simulink model "csc_est_state_estimation_hrn"  (R2014b)
settings: Solver=FixedStepDiscrete  StartTime=t0  StopTime=tFinal  FixedStep=sim_dt  RelTol=1e-3
libraries: util_common_lib x18, util_info_lib x1, csc_est_state_est_mtv_lib x1, csu_cfe_cfe_time_lib x1, converted_pressures_t_hrn_initialization x1, converted_temperatures_t_hrn_initialization x1
settings Model: Creator=escrane  LastModifiedBy=escrane
settings DebuggingCC: UnderspecifiedInitializationDetection=Classic  MergeDetectMultiDrivingBlocksExec=none  InheritedTsInSrcMsg=none

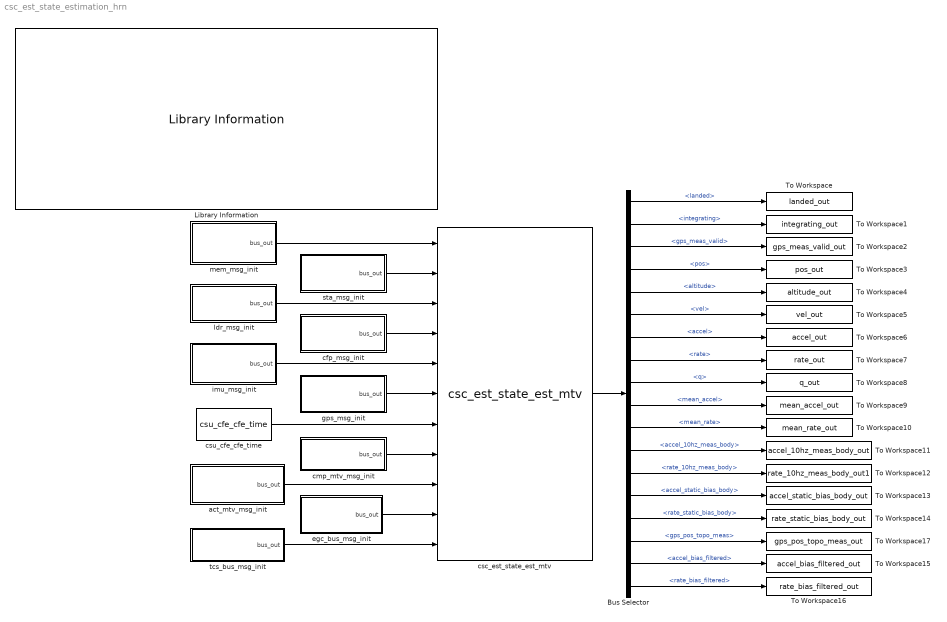
== system csc_est_state_estimation_hrn ==
  Bus Selector : BusSelector  OutputSignals=landed,integrating,gps_meas_valid,pos,altitude,vel,accel,rate,q,mean_accel,mean_rate,accel_10hz_meas_body,rate_10hz_meas_body,accel_static_bias_body,rate_static_bias_body,gps_pos_topo_meas,accel_bias_filtered,rate_bias_filtered
  Library Information : util_info_lib/Library Information  owner='escrane'
  To Workspace : ToWorkspace  VariableName=landed_out  SaveFormat=Timeseries  SampleTime=-1
  To Workspace1 : ToWorkspace  VariableName=integrating_out  SaveFormat=Timeseries  SampleTime=-1
  To Workspace10 : ToWorkspace  VariableName=mean_rate_out  SaveFormat=Timeseries  SampleTime=-1
  To Workspace11 : ToWorkspace  VariableName=accel_10hz_meas_body_out  SaveFormat=Timeseries  SampleTime=-1
  To Workspace12 : ToWorkspace  VariableName=rate_10hz_meas_body_out1  SaveFormat=Timeseries  SampleTime=-1
  To Workspace13 : ToWorkspace  VariableName=accel_static_bias_body_out  SaveFormat=Timeseries  SampleTime=-1
  To Workspace14 : ToWorkspace  VariableName=rate_static_bias_body_out  SaveFormat=Timeseries  SampleTime=-1
  To Workspace15 : ToWorkspace  VariableName=accel_bias_filtered_out  SaveFormat=Timeseries  SampleTime=-1
  To Workspace16 : ToWorkspace  VariableName=rate_bias_filtered_out  SaveFormat=Timeseries  SampleTime=-1
  To Workspace17 : ToWorkspace  VariableName=gps_pos_topo_meas_out  SaveFormat=Timeseries  SampleTime=-1
  To Workspace2 : ToWorkspace  VariableName=gps_meas_valid_out  SaveFormat=Timeseries  SampleTime=-1
  To Workspace3 : ToWorkspace  VariableName=pos_out  SaveFormat=Timeseries  SampleTime=-1
  To Workspace4 : ToWorkspace  VariableName=altitude_out  SaveFormat=Timeseries  SampleTime=-1
  To Workspace5 : ToWorkspace  VariableName=vel_out  SaveFormat=Timeseries  SampleTime=-1
  To Workspace6 : ToWorkspace  VariableName=accel_out  SaveFormat=Timeseries  SampleTime=-1
  To Workspace7 : ToWorkspace  VariableName=rate_out  SaveFormat=Timeseries  SampleTime=-1
  To Workspace8 : ToWorkspace  VariableName=q_out  SaveFormat=Timeseries  SampleTime=-1
  To Workspace9 : ToWorkspace  VariableName=mean_accel_out  SaveFormat=Timeseries  SampleTime=-1
  act_mtv_msg_init : Subsystem
  cfp_msg_init : Subsystem
  cmp_mtv_msg_init : Subsystem
  csc_est_state_est_mtv : csc_est_state_est_mtv_lib/csc_est_state_est_mtv  Tag=OFSW; MDL_TICK=CMP_MTV_MSG
  csu_cfe_cfe_time : csu_cfe_cfe_time_lib/csu_cfe_cfe_time  sch_dt=fsw_dt
  egc_bus_msg_init : Subsystem
  gps_msg_init : Subsystem
  imu_msg_init : Subsystem
  ldr_msg_init : Subsystem
  mem_msg_init : Subsystem
  sta_msg_init : Subsystem
  tcs_bus_msg_init : Subsystem
  wires:
  Bus Selector/1 -> To Workspace/1  "<landed>"
  csc_est_state_est_mtv/1 -> Bus Selector/1
  mem_msg_init/1(bus_out) -> csc_est_state_est_mtv/1
  cmp_mtv_msg_init/1(bus_out) -> csc_est_state_est_mtv/8
  act_mtv_msg_init/1(bus_out) -> csc_est_state_est_mtv/9
  gps_msg_init/1(bus_out) -> csc_est_state_est_mtv/6
  cfp_msg_init/1(bus_out) -> csc_est_state_est_mtv/4
  ldr_msg_init/1(bus_out) -> csc_est_state_est_mtv/3
  sta_msg_init/1(bus_out) -> csc_est_state_est_mtv/2
  csu_cfe_cfe_time/1 -> csc_est_state_est_mtv/7
  Bus Selector/2 -> To Workspace1/1  "<integrating>"
  Bus Selector/3 -> To Workspace2/1  "<gps_meas_valid>"
  Bus Selector/4 -> To Workspace3/1  "<pos>"
  Bus Selector/5 -> To Workspace4/1  "<altitude>"
  Bus Selector/6 -> To Workspace5/1  "<vel>"
  Bus Selector/7 -> To Workspace6/1  "<accel>"
  Bus Selector/8 -> To Workspace7/1  "<rate>"
  Bus Selector/9 -> To Workspace8/1  "<q>"
  Bus Selector/10 -> To Workspace9/1  "<mean_accel>"
  Bus Selector/11 -> To Workspace10/1  "<mean_rate>"
  Bus Selector/12 -> To Workspace11/1  "<accel_10hz_meas_body>"
  Bus Selector/13 -> To Workspace12/1  "<rate_10hz_meas_body>"
  Bus Selector/14 -> To Workspace13/1  "<accel_static_bias_body>"
  Bus Selector/15 -> To Workspace14/1  "<rate_static_bias_body>"
  Bus Selector/18 -> To Workspace16/1  "<rate_bias_filtered>"
  Bus Selector/17 -> To Workspace15/1  "<accel_bias_filtered>"
  Bus Selector/16 -> To Workspace17/1  "<gps_pos_topo_meas>"
  tcs_bus_msg_init/1(bus_out) -> csc_est_state_est_mtv/11
  egc_bus_msg_init/1(bus_out) -> csc_est_state_est_mtv/10
  imu_msg_init/1(bus_out) -> csc_est_state_est_mtv/5

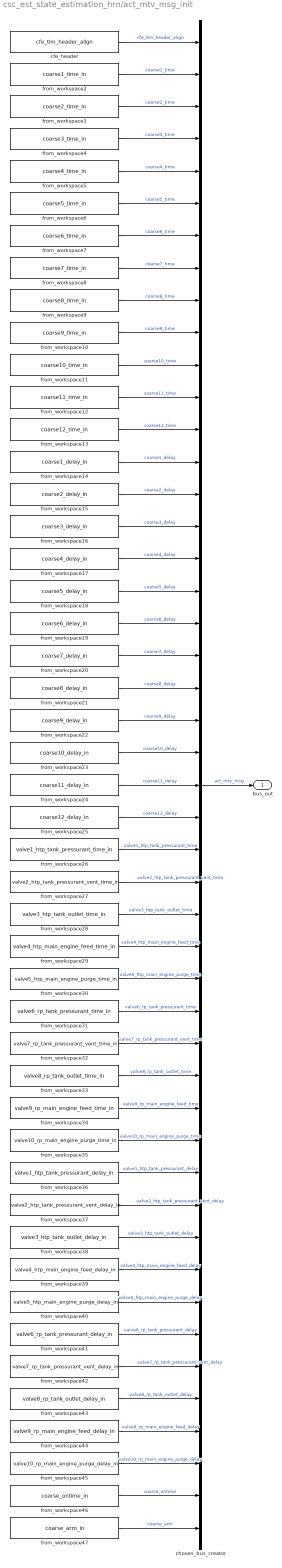
== system csc_est_state_estimation_hrn/act_mtv_msg_init ==
  cfe_header : util_common_lib/cfe_tlm_header_align
  chosen_bus_creator : BusCreator  Inputs=47  OutDataTypeStr=Bus: act_mtv_msg
  from_workspace10 : FromWorkspace  VariableName=coarse9_time_in
  from_workspace11 : FromWorkspace  VariableName=coarse10_time_in
  from_workspace12 : FromWorkspace  VariableName=coarse11_time_in
  from_workspace13 : FromWorkspace  VariableName=coarse12_time_in
  from_workspace14 : FromWorkspace  VariableName=coarse1_delay_in
  from_workspace15 : FromWorkspace  VariableName=coarse2_delay_in
  from_workspace16 : FromWorkspace  VariableName=coarse3_delay_in
  from_workspace17 : FromWorkspace  VariableName=coarse4_delay_in
  from_workspace18 : FromWorkspace  VariableName=coarse5_delay_in
  from_workspace19 : FromWorkspace  VariableName=coarse6_delay_in
  from_workspace2 : FromWorkspace  VariableName=coarse1_time_in
  from_workspace20 : FromWorkspace  VariableName=coarse7_delay_in
  from_workspace21 : FromWorkspace  VariableName=coarse8_delay_in
  from_workspace22 : FromWorkspace  VariableName=coarse9_delay_in
  from_workspace23 : FromWorkspace  VariableName=coarse10_delay_in
  from_workspace24 : FromWorkspace  VariableName=coarse11_delay_in
  from_workspace25 : FromWorkspace  VariableName=coarse12_delay_in
  from_workspace26 : FromWorkspace  VariableName=valve1_htp_tank_pressurant_time_in
  from_workspace27 : FromWorkspace  VariableName=valve2_htp_tank_pressurant_vent_time_in
  from_workspace28 : FromWorkspace  VariableName=valve3_htp_tank_outlet_time_in
  from_workspace29 : FromWorkspace  VariableName=valve4_htp_main_engine_feed_time_in
  from_workspace3 : FromWorkspace  VariableName=coarse2_time_in
  from_workspace30 : FromWorkspace  VariableName=valve5_htp_main_engine_purge_time_in
  from_workspace31 : FromWorkspace  VariableName=valve6_rp_tank_pressurant_time_in
  from_workspace32 : FromWorkspace  VariableName=valve7_rp_tank_pressurant_vent_time_in
  from_workspace33 : FromWorkspace  VariableName=valve8_rp_tank_outlet_time_in
  from_workspace34 : FromWorkspace  VariableName=valve9_rp_main_engine_feed_time_in
  from_workspace35 : FromWorkspace  VariableName=valve10_rp_main_engine_purge_time_in
  from_workspace36 : FromWorkspace  VariableName=valve1_htp_tank_pressurant_delay_in
  from_workspace37 : FromWorkspace  VariableName=valve2_htp_tank_pressurant_vent_delay_in
  from_workspace38 : FromWorkspace  VariableName=valve3_htp_tank_outlet_delay_in
  from_workspace39 : FromWorkspace  VariableName=valve4_htp_main_engine_feed_delay_in
  from_workspace4 : FromWorkspace  VariableName=coarse3_time_in
  from_workspace40 : FromWorkspace  VariableName=valve5_htp_main_engine_purge_delay_in
  from_workspace41 : FromWorkspace  VariableName=valve6_rp_tank_pressurant_delay_in
  from_workspace42 : FromWorkspace  VariableName=valve7_rp_tank_pressurant_vent_delay_in
  from_workspace43 : FromWorkspace  VariableName=valve8_rp_tank_outlet_delay_in
  from_workspace44 : FromWorkspace  VariableName=valve9_rp_main_engine_feed_delay_in
  from_workspace45 : FromWorkspace  VariableName=valve10_rp_main_engine_purge_delay_in
  from_workspace46 : FromWorkspace  VariableName=coarse_ontime_in
  from_workspace47 : FromWorkspace  VariableName=coarse_arm_in
  from_workspace5 : FromWorkspace  VariableName=coarse4_time_in
  from_workspace6 : FromWorkspace  VariableName=coarse5_time_in
  from_workspace7 : FromWorkspace  VariableName=coarse6_time_in
  from_workspace8 : FromWorkspace  VariableName=coarse7_time_in
  from_workspace9 : FromWorkspace  VariableName=coarse8_time_in
  bus_out : Outport
  wires:
  from_workspace47/1 -> chosen_bus_creator/47  "coarse_arm"
  from_workspace46/1 -> chosen_bus_creator/46  "coarse_ontime"
  from_workspace45/1 -> chosen_bus_creator/45  "valve10_rp_main_engine_purge_delay"
  from_workspace44/1 -> chosen_bus_creator/44  "valve9_rp_main_engine_feed_delay"
  from_workspace43/1 -> chosen_bus_creator/43  "valve8_rp_tank_outlet_delay"
  from_workspace42/1 -> chosen_bus_creator/42  "valve7_rp_tank_pressurant_vent_delay"
  from_workspace41/1 -> chosen_bus_creator/41  "valve6_rp_tank_pressurant_delay"
  from_workspace40/1 -> chosen_bus_creator/40  "valve5_htp_main_engine_purge_delay"
  from_workspace39/1 -> chosen_bus_creator/39  "valve4_htp_main_engine_feed_delay"
  from_workspace38/1 -> chosen_bus_creator/38  "valve3_htp_tank_outlet_delay"
  from_workspace37/1 -> chosen_bus_creator/37  "valve2_htp_tank_pressurant_vent_delay"
  from_workspace36/1 -> chosen_bus_creator/36  "valve1_htp_tank_pressurant_delay"
  from_workspace35/1 -> chosen_bus_creator/35  "valve10_rp_main_engine_purge_time"
  from_workspace34/1 -> chosen_bus_creator/34  "valve9_rp_main_engine_feed_time"
  from_workspace33/1 -> chosen_bus_creator/33  "valve8_rp_tank_outlet_time"
  from_workspace32/1 -> chosen_bus_creator/32  "valve7_rp_tank_pressurant_vent_time"
  from_workspace31/1 -> chosen_bus_creator/31  "valve6_rp_tank_pressurant_time"
  from_workspace30/1 -> chosen_bus_creator/30  "valve5_htp_main_engine_purge_time"
  from_workspace29/1 -> chosen_bus_creator/29  "valve4_htp_main_engine_feed_time"
  from_workspace28/1 -> chosen_bus_creator/28  "valve3_htp_tank_outlet_time"
  from_workspace27/1 -> chosen_bus_creator/27  "valve2_htp_tank_pressurant_vent_time"
  from_workspace26/1 -> chosen_bus_creator/26  "valve1_htp_tank_pressurant_time"
  from_workspace25/1 -> chosen_bus_creator/25  "coarse12_delay"
  from_workspace24/1 -> chosen_bus_creator/24  "coarse11_delay"
  from_workspace23/1 -> chosen_bus_creator/23  "coarse10_delay"
  from_workspace22/1 -> chosen_bus_creator/22  "coarse9_delay"
  from_workspace21/1 -> chosen_bus_creator/21  "coarse8_delay"
  from_workspace20/1 -> chosen_bus_creator/20  "coarse7_delay"
  from_workspace19/1 -> chosen_bus_creator/19  "coarse6_delay"
  from_workspace18/1 -> chosen_bus_creator/18  "coarse5_delay"
  from_workspace17/1 -> chosen_bus_creator/17  "coarse4_delay"
  from_workspace16/1 -> chosen_bus_creator/16  "coarse3_delay"
  from_workspace15/1 -> chosen_bus_creator/15  "coarse2_delay"
  from_workspace14/1 -> chosen_bus_creator/14  "coarse1_delay"
  from_workspace13/1 -> chosen_bus_creator/13  "coarse12_time"
  from_workspace12/1 -> chosen_bus_creator/12  "coarse11_time"
  from_workspace11/1 -> chosen_bus_creator/11  "coarse10_time"
  from_workspace10/1 -> chosen_bus_creator/10  "coarse9_time"
  from_workspace9/1 -> chosen_bus_creator/9  "coarse8_time"
  from_workspace8/1 -> chosen_bus_creator/8  "coarse7_time"
  from_workspace7/1 -> chosen_bus_creator/7  "coarse6_time"
  from_workspace6/1 -> chosen_bus_creator/6  "coarse5_time"
  from_workspace5/1 -> chosen_bus_creator/5  "coarse4_time"
  from_workspace4/1 -> chosen_bus_creator/4  "coarse3_time"
  from_workspace3/1 -> chosen_bus_creator/3  "coarse2_time"
  from_workspace2/1 -> chosen_bus_creator/2  "coarse1_time"
  cfe_header/1 -> chosen_bus_creator/1  "cfe_tlm_header_align"
  chosen_bus_creator/1 -> bus_out/1  "act_mtv_msg"

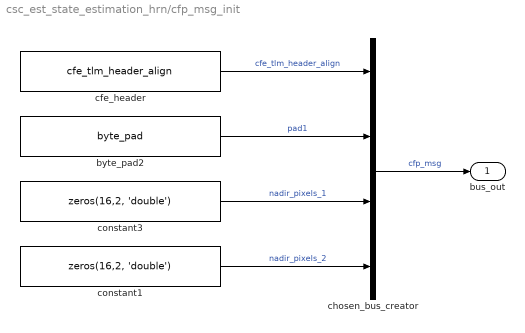
== system csc_est_state_estimation_hrn/cfp_msg_init ==
  byte_pad2 : util_common_lib/byte_pad  n_bytes=4
  cfe_header : util_common_lib/cfe_tlm_header_align
  chosen_bus_creator : BusCreator  OutDataTypeStr=Bus: cfp_msg  NonVirtualBus=on
  constant1 : Constant  Value=zeros(16,2, 'double')
  constant3 : Constant  Value=zeros(16,2, 'double')
  bus_out : Outport
  wires:
  constant1/1 -> chosen_bus_creator/4  "nadir_pixels_2"
  constant3/1 -> chosen_bus_creator/3  "nadir_pixels_1"
  byte_pad2/1 -> chosen_bus_creator/2  "pad1"
  cfe_header/1 -> chosen_bus_creator/1  "cfe_tlm_header_align"
  chosen_bus_creator/1 -> bus_out/1  "cfp_msg"

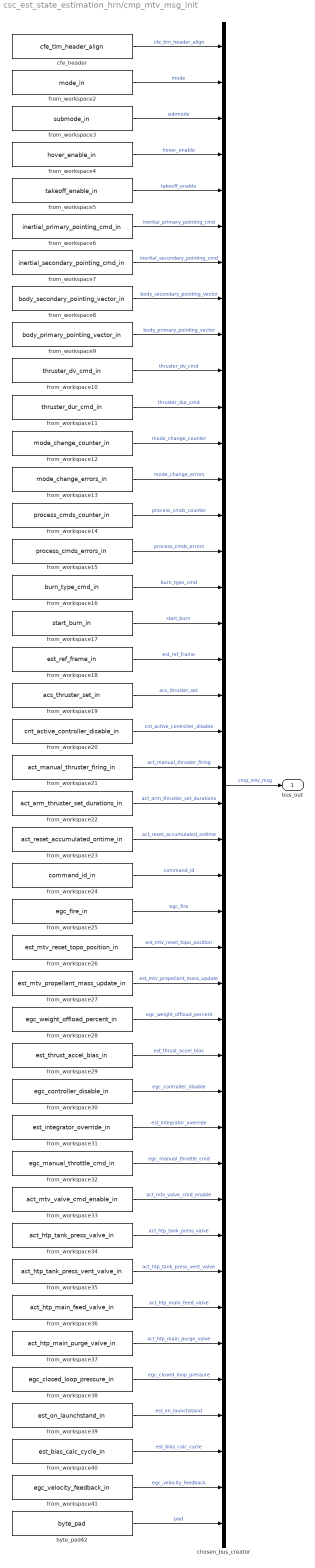
== system csc_est_state_estimation_hrn/cmp_mtv_msg_init ==
  byte_pad42 : util_common_lib/byte_pad  n_bytes=1
  cfe_header : util_common_lib/cfe_tlm_header_align
  chosen_bus_creator : BusCreator  Inputs=42  OutDataTypeStr=Bus: cmp_mtv_msg  NonVirtualBus=on
  from_workspace10 : FromWorkspace  VariableName=thruster_dv_cmd_in
  from_workspace11 : FromWorkspace  VariableName=thruster_dur_cmd_in
  from_workspace12 : FromWorkspace  VariableName=mode_change_counter_in
  from_workspace13 : FromWorkspace  VariableName=mode_change_errors_in
  from_workspace14 : FromWorkspace  VariableName=process_cmds_counter_in
  from_workspace15 : FromWorkspace  VariableName=process_cmds_errors_in
  from_workspace16 : FromWorkspace  VariableName=burn_type_cmd_in
  from_workspace17 : FromWorkspace  VariableName=start_burn_in
  from_workspace18 : FromWorkspace  VariableName=est_ref_frame_in
  from_workspace19 : FromWorkspace  VariableName=acs_thruster_set_in
  from_workspace2 : FromWorkspace  VariableName=mode_in
  from_workspace20 : FromWorkspace  VariableName=cnt_active_controller_disable_in
  from_workspace21 : FromWorkspace  VariableName=act_manual_thruster_firing_in
  from_workspace22 : FromWorkspace  VariableName=act_arm_thruster_set_durations_in
  from_workspace23 : FromWorkspace  VariableName=act_reset_accumulated_ontime_in
  from_workspace24 : FromWorkspace  VariableName=command_id_in
  from_workspace25 : FromWorkspace  VariableName=egc_fire_in
  from_workspace26 : FromWorkspace  VariableName=est_mtv_reset_topo_position_in
  from_workspace27 : FromWorkspace  VariableName=est_mtv_propellant_mass_update_in
  from_workspace28 : FromWorkspace  VariableName=egc_weight_offload_percent_in
  from_workspace29 : FromWorkspace  VariableName=est_thrust_accel_bias_in
  from_workspace3 : FromWorkspace  VariableName=submode_in
  from_workspace30 : FromWorkspace  VariableName=egc_controller_disable_in
  from_workspace31 : FromWorkspace  VariableName=est_integrator_override_in
  from_workspace32 : FromWorkspace  VariableName=egc_manual_throttle_cmd_in
  from_workspace33 : FromWorkspace  VariableName=act_mtv_valve_cmd_enable_in
  from_workspace34 : FromWorkspace  VariableName=act_htp_tank_press_valve_in
  from_workspace35 : FromWorkspace  VariableName=act_htp_tank_press_vent_valve_in
  from_workspace36 : FromWorkspace  VariableName=act_htp_main_feed_valve_in
  from_workspace37 : FromWorkspace  VariableName=act_htp_main_purge_valve_in
  from_workspace38 : FromWorkspace  VariableName=egc_closed_loop_pressure_in
  from_workspace39 : FromWorkspace  VariableName=est_on_launchstand_in
  from_workspace4 : FromWorkspace  VariableName=hover_enable_in
  from_workspace40 : FromWorkspace  VariableName=est_bias_calc_cycle_in
  from_workspace41 : FromWorkspace  VariableName=egc_velocity_feedback_in
  from_workspace5 : FromWorkspace  VariableName=takeoff_enable_in
  from_workspace6 : FromWorkspace  VariableName=inertial_primary_pointing_cmd_in
  from_workspace7 : FromWorkspace  VariableName=inertial_secondary_pointing_cmd_in
  from_workspace8 : FromWorkspace  VariableName=body_secondary_pointing_vector_in
  from_workspace9 : FromWorkspace  VariableName=body_primary_pointing_vector_in
  bus_out : Outport
  wires:
  byte_pad42/1 -> chosen_bus_creator/42  "pad"
  from_workspace41/1 -> chosen_bus_creator/41  "egc_velocity_feedback"
  from_workspace40/1 -> chosen_bus_creator/40  "est_bias_calc_cycle"
  from_workspace39/1 -> chosen_bus_creator/39  "est_on_launchstand"
  from_workspace38/1 -> chosen_bus_creator/38  "egc_closed_loop_pressure"
  from_workspace37/1 -> chosen_bus_creator/37  "act_htp_main_purge_valve"
  from_workspace36/1 -> chosen_bus_creator/36  "act_htp_main_feed_valve"
  from_workspace35/1 -> chosen_bus_creator/35  "act_htp_tank_press_vent_valve"
  from_workspace34/1 -> chosen_bus_creator/34  "act_htp_tank_press_valve"
  from_workspace33/1 -> chosen_bus_creator/33  "act_mtv_valve_cmd_enable"
  from_workspace32/1 -> chosen_bus_creator/32  "egc_manual_throttle_cmd"
  from_workspace31/1 -> chosen_bus_creator/31  "est_integrator_override"
  from_workspace30/1 -> chosen_bus_creator/30  "egc_controller_disable"
  from_workspace29/1 -> chosen_bus_creator/29  "est_thrust_accel_bias"
  from_workspace28/1 -> chosen_bus_creator/28  "egc_weight_offload_percent"
  from_workspace27/1 -> chosen_bus_creator/27  "est_mtv_propellant_mass_update"
  from_workspace26/1 -> chosen_bus_creator/26  "est_mtv_reset_topo_position"
  from_workspace25/1 -> chosen_bus_creator/25  "egc_fire"
  from_workspace24/1 -> chosen_bus_creator/24  "command_id"
  from_workspace23/1 -> chosen_bus_creator/23  "act_reset_accumulated_ontime"
  from_workspace22/1 -> chosen_bus_creator/22  "act_arm_thruster_set_durations"
  from_workspace21/1 -> chosen_bus_creator/21  "act_manual_thruster_firing"
  from_workspace20/1 -> chosen_bus_creator/20  "cnt_active_controller_disable"
  from_workspace19/1 -> chosen_bus_creator/19  "acs_thruster_set"
  from_workspace18/1 -> chosen_bus_creator/18  "est_ref_frame"
  from_workspace17/1 -> chosen_bus_creator/17  "start_burn"
  from_workspace16/1 -> chosen_bus_creator/16  "burn_type_cmd"
  from_workspace15/1 -> chosen_bus_creator/15  "process_cmds_errors"
  from_workspace14/1 -> chosen_bus_creator/14  "process_cmds_counter"
  from_workspace13/1 -> chosen_bus_creator/13  "mode_change_errors"
  from_workspace12/1 -> chosen_bus_creator/12  "mode_change_counter"
  from_workspace11/1 -> chosen_bus_creator/11  "thruster_dur_cmd"
  from_workspace10/1 -> chosen_bus_creator/10  "thruster_dv_cmd"
  from_workspace9/1 -> chosen_bus_creator/9  "body_primary_pointing_vector"
  from_workspace8/1 -> chosen_bus_creator/8  "body_secondary_pointing_vector"
  from_workspace7/1 -> chosen_bus_creator/7  "inertial_secondary_pointing_cmd"
  from_workspace6/1 -> chosen_bus_creator/6  "inertial_primary_pointing_cmd"
  from_workspace5/1 -> chosen_bus_creator/5  "takeoff_enable"
  from_workspace4/1 -> chosen_bus_creator/4  "hover_enable"
  from_workspace3/1 -> chosen_bus_creator/3  "submode"
  from_workspace2/1 -> chosen_bus_creator/2  "mode"
  cfe_header/1 -> chosen_bus_creator/1  "cfe_tlm_header_align"
  chosen_bus_creator/1 -> bus_out/1  "cmp_mtv_msg"

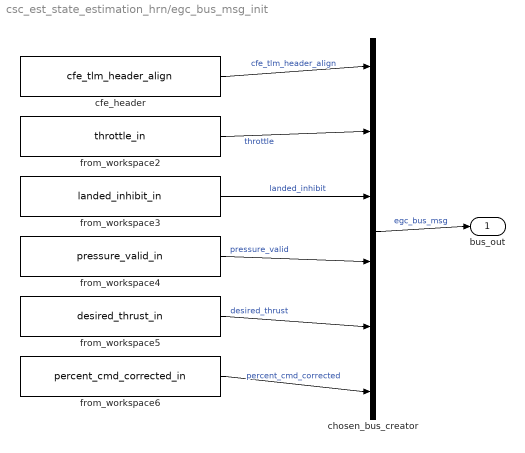
== system csc_est_state_estimation_hrn/egc_bus_msg_init ==
  cfe_header : util_common_lib/cfe_tlm_header_align
  chosen_bus_creator : BusCreator  Inputs=6  OutDataTypeStr=Bus: egc_bus_msg  NonVirtualBus=on
  from_workspace2 : FromWorkspace  VariableName=throttle_in
  from_workspace3 : FromWorkspace  VariableName=landed_inhibit_in
  from_workspace4 : FromWorkspace  VariableName=pressure_valid_in
  from_workspace5 : FromWorkspace  VariableName=desired_thrust_in
  from_workspace6 : FromWorkspace  VariableName=percent_cmd_corrected_in
  bus_out : Outport
  wires:
  from_workspace6/1 -> chosen_bus_creator/6  "percent_cmd_corrected"
  from_workspace5/1 -> chosen_bus_creator/5  "desired_thrust"
  from_workspace4/1 -> chosen_bus_creator/4  "pressure_valid"
  from_workspace3/1 -> chosen_bus_creator/3  "landed_inhibit"
  from_workspace2/1 -> chosen_bus_creator/2  "throttle"
  cfe_header/1 -> chosen_bus_creator/1  "cfe_tlm_header_align"
  chosen_bus_creator/1 -> bus_out/1  "egc_bus_msg"

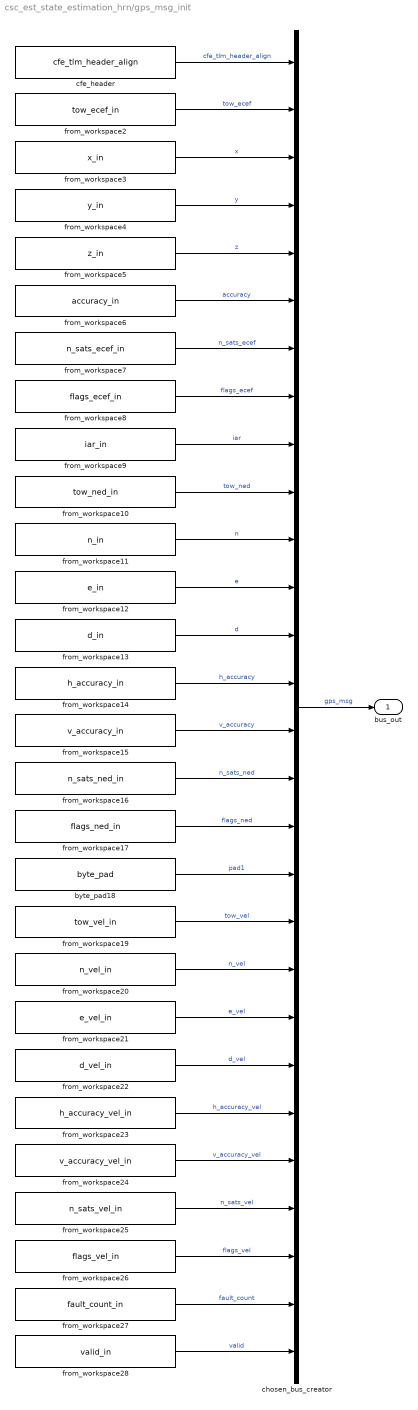
== system csc_est_state_estimation_hrn/gps_msg_init ==
  byte_pad18 : util_common_lib/byte_pad  n_bytes=2
  cfe_header : util_common_lib/cfe_tlm_header_align
  chosen_bus_creator : BusCreator  Inputs=28  OutDataTypeStr=Bus: gps_msg  NonVirtualBus=on
  from_workspace10 : FromWorkspace  VariableName=tow_ned_in
  from_workspace11 : FromWorkspace  VariableName=n_in
  from_workspace12 : FromWorkspace  VariableName=e_in
  from_workspace13 : FromWorkspace  VariableName=d_in
  from_workspace14 : FromWorkspace  VariableName=h_accuracy_in
  from_workspace15 : FromWorkspace  VariableName=v_accuracy_in
  from_workspace16 : FromWorkspace  VariableName=n_sats_ned_in
  from_workspace17 : FromWorkspace  VariableName=flags_ned_in
  from_workspace19 : FromWorkspace  VariableName=tow_vel_in
  from_workspace2 : FromWorkspace  VariableName=tow_ecef_in
  from_workspace20 : FromWorkspace  VariableName=n_vel_in
  from_workspace21 : FromWorkspace  VariableName=e_vel_in
  from_workspace22 : FromWorkspace  VariableName=d_vel_in
  from_workspace23 : FromWorkspace  VariableName=h_accuracy_vel_in
  from_workspace24 : FromWorkspace  VariableName=v_accuracy_vel_in
  from_workspace25 : FromWorkspace  VariableName=n_sats_vel_in
  from_workspace26 : FromWorkspace  VariableName=flags_vel_in
  from_workspace27 : FromWorkspace  VariableName=fault_count_in
  from_workspace28 : FromWorkspace  VariableName=valid_in
  from_workspace3 : FromWorkspace  VariableName=x_in
  from_workspace4 : FromWorkspace  VariableName=y_in
  from_workspace5 : FromWorkspace  VariableName=z_in
  from_workspace6 : FromWorkspace  VariableName=accuracy_in
  from_workspace7 : FromWorkspace  VariableName=n_sats_ecef_in
  from_workspace8 : FromWorkspace  VariableName=flags_ecef_in
  from_workspace9 : FromWorkspace  VariableName=iar_in
  bus_out : Outport
  wires:
  from_workspace28/1 -> chosen_bus_creator/28  "valid"
  from_workspace27/1 -> chosen_bus_creator/27  "fault_count"
  from_workspace26/1 -> chosen_bus_creator/26  "flags_vel"
  from_workspace25/1 -> chosen_bus_creator/25  "n_sats_vel"
  from_workspace24/1 -> chosen_bus_creator/24  "v_accuracy_vel"
  from_workspace23/1 -> chosen_bus_creator/23  "h_accuracy_vel"
  from_workspace22/1 -> chosen_bus_creator/22  "d_vel"
  from_workspace21/1 -> chosen_bus_creator/21  "e_vel"
  from_workspace20/1 -> chosen_bus_creator/20  "n_vel"
  from_workspace19/1 -> chosen_bus_creator/19  "tow_vel"
  byte_pad18/1 -> chosen_bus_creator/18  "pad1"
  from_workspace17/1 -> chosen_bus_creator/17  "flags_ned"
  from_workspace16/1 -> chosen_bus_creator/16  "n_sats_ned"
  from_workspace15/1 -> chosen_bus_creator/15  "v_accuracy"
  from_workspace14/1 -> chosen_bus_creator/14  "h_accuracy"
  from_workspace13/1 -> chosen_bus_creator/13  "d"
  from_workspace12/1 -> chosen_bus_creator/12  "e"
  from_workspace11/1 -> chosen_bus_creator/11  "n"
  from_workspace10/1 -> chosen_bus_creator/10  "tow_ned"
  from_workspace9/1 -> chosen_bus_creator/9  "iar"
  from_workspace8/1 -> chosen_bus_creator/8  "flags_ecef"
  from_workspace7/1 -> chosen_bus_creator/7  "n_sats_ecef"
  from_workspace6/1 -> chosen_bus_creator/6  "accuracy"
  from_workspace5/1 -> chosen_bus_creator/5  "z"
  from_workspace4/1 -> chosen_bus_creator/4  "y"
  from_workspace3/1 -> chosen_bus_creator/3  "x"
  from_workspace2/1 -> chosen_bus_creator/2  "tow_ecef"
  cfe_header/1 -> chosen_bus_creator/1  "cfe_tlm_header_align"
  chosen_bus_creator/1 -> bus_out/1  "gps_msg"

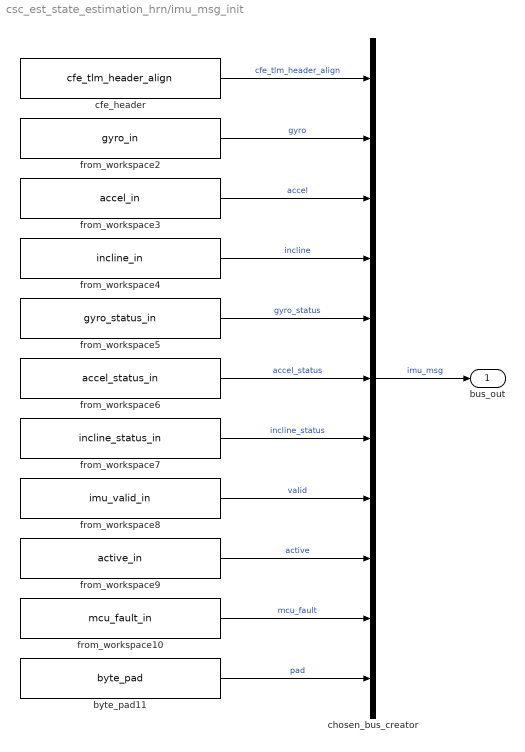
== system csc_est_state_estimation_hrn/imu_msg_init ==
  byte_pad11 : util_common_lib/byte_pad  n_bytes=2
  cfe_header : util_common_lib/cfe_tlm_header_align
  chosen_bus_creator : BusCreator  Inputs=11  OutDataTypeStr=Bus: imu_msg  NonVirtualBus=on
  from_workspace10 : FromWorkspace  VariableName=mcu_fault_in
  from_workspace2 : FromWorkspace  VariableName=gyro_in
  from_workspace3 : FromWorkspace  VariableName=accel_in
  from_workspace4 : FromWorkspace  VariableName=incline_in
  from_workspace5 : FromWorkspace  VariableName=gyro_status_in
  from_workspace6 : FromWorkspace  VariableName=accel_status_in
  from_workspace7 : FromWorkspace  VariableName=incline_status_in
  from_workspace8 : FromWorkspace  VariableName=imu_valid_in
  from_workspace9 : FromWorkspace  VariableName=active_in
  bus_out : Outport
  wires:
  byte_pad11/1 -> chosen_bus_creator/11  "pad"
  from_workspace10/1 -> chosen_bus_creator/10  "mcu_fault"
  from_workspace9/1 -> chosen_bus_creator/9  "active"
  from_workspace8/1 -> chosen_bus_creator/8  "valid"
  from_workspace7/1 -> chosen_bus_creator/7  "incline_status"
  from_workspace6/1 -> chosen_bus_creator/6  "accel_status"
  from_workspace5/1 -> chosen_bus_creator/5  "gyro_status"
  from_workspace4/1 -> chosen_bus_creator/4  "incline"
  from_workspace3/1 -> chosen_bus_creator/3  "accel"
  from_workspace2/1 -> chosen_bus_creator/2  "gyro"
  cfe_header/1 -> chosen_bus_creator/1  "cfe_tlm_header_align"
  chosen_bus_creator/1 -> bus_out/1  "imu_msg"

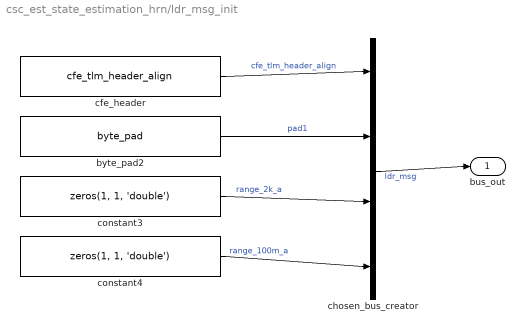
== system csc_est_state_estimation_hrn/ldr_msg_init ==
  byte_pad2 : util_common_lib/byte_pad  n_bytes=4
  cfe_header : util_common_lib/cfe_tlm_header_align
  chosen_bus_creator : BusCreator  OutDataTypeStr=Bus: ldr_msg  NonVirtualBus=on
  constant3 : Constant  Value=zeros(1, 1, 'double')
  constant4 : Constant  Value=zeros(1, 1, 'double')
  bus_out : Outport
  wires:
  constant4/1 -> chosen_bus_creator/4  "range_100m_a"
  constant3/1 -> chosen_bus_creator/3  "range_2k_a"
  byte_pad2/1 -> chosen_bus_creator/2  "pad1"
  cfe_header/1 -> chosen_bus_creator/1  "cfe_tlm_header_align"
  chosen_bus_creator/1 -> bus_out/1  "ldr_msg"

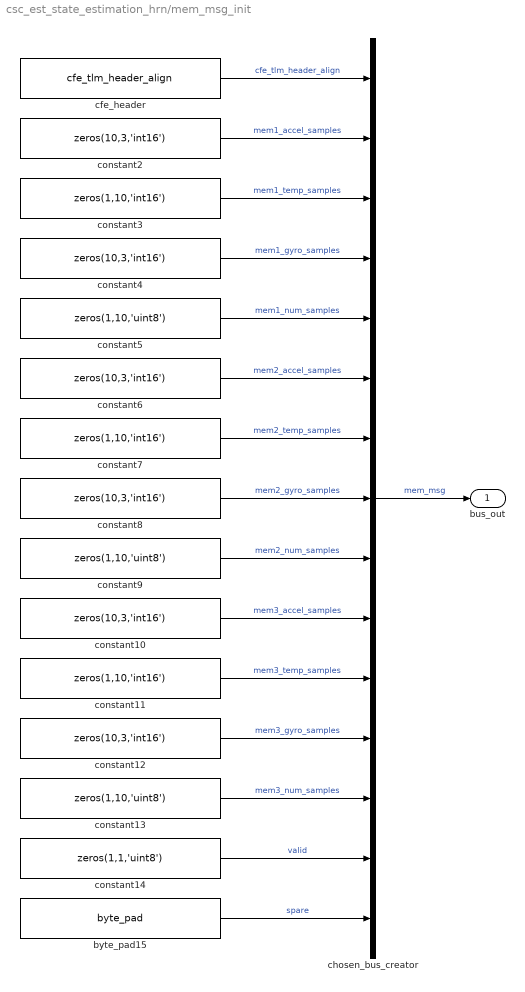
== system csc_est_state_estimation_hrn/mem_msg_init ==
  byte_pad15 : util_common_lib/byte_pad  n_bytes=1
  cfe_header : util_common_lib/cfe_tlm_header_align
  chosen_bus_creator : BusCreator  Inputs=15  OutDataTypeStr=Bus: mem_msg  NonVirtualBus=on
  constant{2,4,6,8,10,12} (6 alike) : Constant  Value=zeros(10,3,'int16')
  constant11 : Constant  Value=zeros(1,10,'int16')
  constant13 : Constant  Value=zeros(1,10,'uint8')
  constant14 : Constant  Value=zeros(1,1,'uint8')
  constant3 : Constant  Value=zeros(1,10,'int16')
  constant5 : Constant  Value=zeros(1,10,'uint8')
  constant7 : Constant  Value=zeros(1,10,'int16')
  constant9 : Constant  Value=zeros(1,10,'uint8')
  bus_out : Outport
  wires:
  byte_pad15/1 -> chosen_bus_creator/15  "spare"
  constant14/1 -> chosen_bus_creator/14  "valid"
  constant13/1 -> chosen_bus_creator/13  "mem3_num_samples"
  constant12/1 -> chosen_bus_creator/12  "mem3_gyro_samples"
  constant11/1 -> chosen_bus_creator/11  "mem3_temp_samples"
  constant10/1 -> chosen_bus_creator/10  "mem3_accel_samples"
  constant9/1 -> chosen_bus_creator/9  "mem2_num_samples"
  constant8/1 -> chosen_bus_creator/8  "mem2_gyro_samples"
  constant7/1 -> chosen_bus_creator/7  "mem2_temp_samples"
  constant6/1 -> chosen_bus_creator/6  "mem2_accel_samples"
  constant5/1 -> chosen_bus_creator/5  "mem1_num_samples"
  constant4/1 -> chosen_bus_creator/4  "mem1_gyro_samples"
  constant3/1 -> chosen_bus_creator/3  "mem1_temp_samples"
  constant2/1 -> chosen_bus_creator/2  "mem1_accel_samples"
  cfe_header/1 -> chosen_bus_creator/1  "cfe_tlm_header_align"
  chosen_bus_creator/1 -> bus_out/1  "mem_msg"

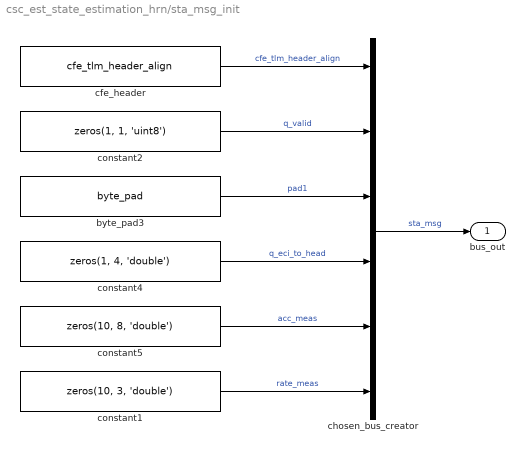
== system csc_est_state_estimation_hrn/sta_msg_init ==
  byte_pad3 : util_common_lib/byte_pad  n_bytes=3
  cfe_header : util_common_lib/cfe_tlm_header_align
  chosen_bus_creator : BusCreator  Inputs=6  OutDataTypeStr=Bus: sta_msg  NonVirtualBus=on
  constant1 : Constant  Value=zeros(10, 3, 'double')
  constant2 : Constant  Value=zeros(1, 1, 'uint8')
  constant4 : Constant  Value=zeros(1, 4, 'double')
  constant5 : Constant  Value=zeros(10, 8, 'double')
  bus_out : Outport
  wires:
  constant1/1 -> chosen_bus_creator/6  "rate_meas"
  constant5/1 -> chosen_bus_creator/5  "acc_meas"
  constant4/1 -> chosen_bus_creator/4  "q_eci_to_head"
  byte_pad3/1 -> chosen_bus_creator/3  "pad1"
  constant2/1 -> chosen_bus_creator/2  "q_valid"
  cfe_header/1 -> chosen_bus_creator/1  "cfe_tlm_header_align"
  chosen_bus_creator/1 -> bus_out/1  "sta_msg"

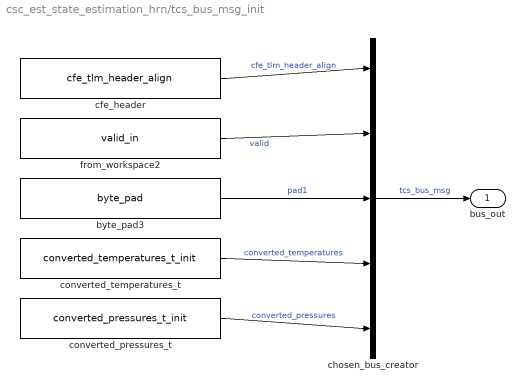
== system csc_est_state_estimation_hrn/tcs_bus_msg_init ==
  byte_pad3 : util_common_lib/byte_pad  n_bytes=7
  cfe_header : util_common_lib/cfe_tlm_header_align
  chosen_bus_creator : BusCreator  Inputs=5  OutDataTypeStr=Bus: tcs_bus_msg  NonVirtualBus=on
  converted_pressures_t : converted_pressures_t_hrn_initialization/converted_pressures_t_init
  converted_temperatures_t : converted_temperatures_t_hrn_initialization/converted_temperatures_t_init
  from_workspace2 : FromWorkspace  VariableName=valid_in
  bus_out : Outport
  wires:
  converted_pressures_t/1 -> chosen_bus_creator/5  "converted_pressures"
  converted_temperatures_t/1 -> chosen_bus_creator/4  "converted_temperatures"
  byte_pad3/1 -> chosen_bus_creator/3  "pad1"
  from_workspace2/1 -> chosen_bus_creator/2  "valid"
  cfe_header/1 -> chosen_bus_creator/1  "cfe_tlm_header_align"
  chosen_bus_creator/1 -> bus_out/1  "tcs_bus_msg"
